simulink model "tanqueNL"  (R2018b)
settings: Solver=VariableStepAuto  StartTime=0.0  StopTime=500  RelTol=1e-3
values from neighbouring files (symbols this model uses):
  h1 = h1_ruido(1:end-1)    [Atividade3.m]    (also in ssTanque.m)
  h2 = h2_ruido(1:end-1)    [Atividade3.m]    (also in ssTanque.m)
  k1 = 25    [dadosTanque.m]
  k2 = 25    [dadosTanque.m]
  kac = 20    [dadosTanque.m]
undefined symbols (not defined in the file or in its folder): qin1, qin2
settings Model: Creator=Caléo  LastModifiedBy=Caléo

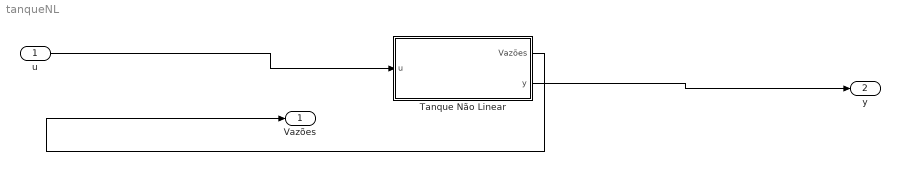
== system tanqueNL ==
  u : Inport
  Tanque Não Linear : Subsystem
  Vazões : Outport
  y : Outport  Port=2
  wires:
  u/1 -> Tanque Não Linear/1(u)
  Tanque Não Linear/1(Vazões) -> Vazões/1
  Tanque Não Linear/2(y) -> y/1

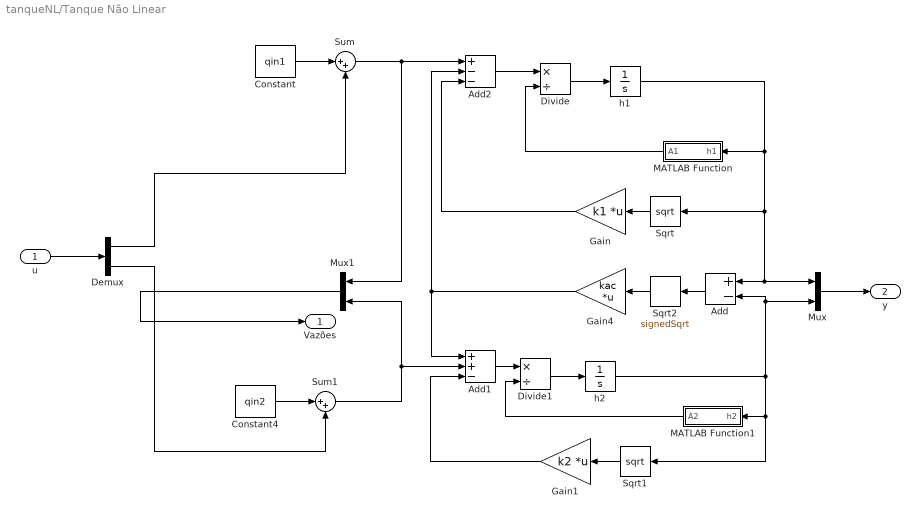
== system tanqueNL/Tanque Não Linear ==
  u : Inport
  Add : Sum  Inputs=+-
  Add1 : Sum  Inputs=++-
  Add2 : Sum  Inputs=+--
  Constant : Constant  Value=qin1
  Constant4 : Constant  Value=qin2
  Demux : Demux  Outputs=2
  Divide : Product  Inputs=*/
  Divide1 : Product  Inputs=*/
  Gain : Gain  Gain=k1  Multiplication=Matrix(K*u)
  Gain1 : Gain  Gain=k2  Multiplication=Matrix(K*u)
  Gain4 : Gain  Gain=kac  Multiplication=Matrix(K*u)
  MATLAB Function : MATLAB Function  TreatAsAtomicUnit=on
  MATLAB Function1 : MATLAB Function  TreatAsAtomicUnit=on
  Mux : Mux  Inputs=2
  Mux1 : Mux  Inputs=2
  Sqrt : Sqrt  SaturateOnIntegerOverflow=on
  Sqrt1 : Sqrt  SaturateOnIntegerOverflow=on
  Sqrt2 : Sqrt  Operator=signedSqrt  SaturateOnIntegerOverflow=on
  Sum : Sum  Inputs=|++
  Sum1 : Sum  Inputs=|++
  h1 : Integrator  InitialCondition=h1  LimitOutput=on  UpperSaturationLimit=50  LowerSaturationLimit=0
  h2 : Integrator  InitialCondition=h2  LimitOutput=on  UpperSaturationLimit=50  LowerSaturationLimit=0
  Vazões : Outport
  y : Outport  Port=2
  wires:
  u/1 -> Demux/1
  h2/1 -> Add/2, Mux/2, MATLAB Function1/1(h2), Sqrt1/1
  Sum/1 -> Mux1/1, Add2/1
  Sum1/1 -> Mux1/2, Add1/2
  Sqrt2/1 -> Gain4/1
  Gain/1 -> Add2/3
  Demux/1 -> Sum/2
  Demux/2 -> Sum1/2
  Divide/1 -> h1/1
  h1/1 -> Mux/1, Add/1, Sqrt/1, MATLAB Function/1(h1)
  Add/1 -> Sqrt2/1
  Mux1/1 -> Vazões/1
  Gain4/1 -> Add2/2, Add1/1
  Sqrt1/1 -> Gain1/1
  Constant/1 -> Sum/1
  Divide1/1 -> h2/1
  Constant4/1 -> Sum1/1
  Add1/1 -> Divide1/1
  MATLAB Function1/1(A2) -> Divide1/2
  Add2/1 -> Divide/1
  MATLAB Function/1(A1) -> Divide/2
  Gain1/1 -> Add1/3
  Mux/1 -> y/1
  Sqrt/1 -> Gain/1

== matlab function tanqueNL/Tanque Não Linear/MATLAB Function1 ==
  data: h2 input; A2 output
function A2 = secao_tanque(h2)

    if h2 < 7.5
        d2 = 6; 
    elseif h2 < 19.5
        d2 = (19.5 - h2)/2;
    elseif h2 < 29.5
        d2 = 0;
    elseif h2 < 41.5
        d2=(h2 - 29.5)/2;
    elseif h2 >= 41.5
        d2 = 6;
    else 
        d2 = 6;
    end
    A2 = 9*(14+d2);
    
end

== matlab function tanqueNL/Tanque Não Linear/MATLAB Function ==
  data: h1 input; A1 output
function A1 = secao_tanque(h1)

    if h1 < 7.5
        d1 = 0;
    elseif h1 < 19.5
        d1 = (h1 - 7.5)/2;
    elseif h1 < 29.5
        d1 = 6;
    elseif h1 < 41.5
        d1 = (41.5 - h1)/2;
    elseif h1 >= 41.5
        d1 = 0;
    else 
        d1 = 0;
    end
    A1 = 9*(8+d1);
end
